simulink model "Quadrotor_1"  (R2018a)
settings: Solver=VariableStepAuto  StartTime=0.0  StopTime=100  MaxStep=0.001  RelTol=1e-3
settings Model: Creator=oussa  LastModifiedBy=oussa

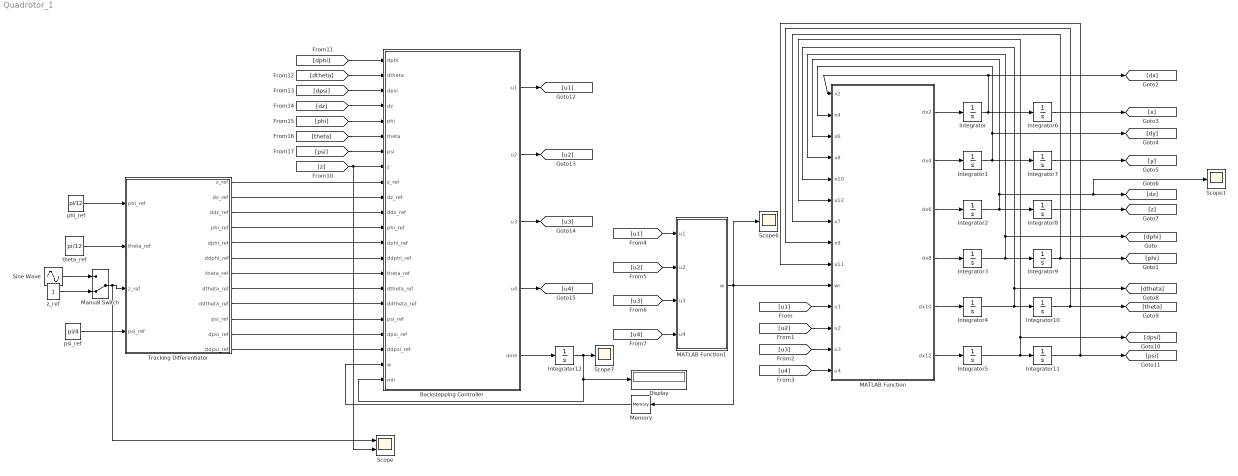
== system Quadrotor_1 ==
  Backstepping Controller : MATLAB Function  TreatAsAtomicUnit=on
  Display : Display
  Integrator{,1..11} (12 alike) : Integrator
  Integrator12 : Integrator  InitialCondition=0.01
  MATLAB Function : MATLAB Function  TreatAsAtomicUnit=on
  MATLAB Function1 : MATLAB Function  TreatAsAtomicUnit=on
  Manual Switch : ManualSwitch  CurrentSetting=0
  Memory : Memory  InitialCondition=500
  Scope : Scope  NumInputPorts=2
  Scope1 : Scope
  Scope6 : Scope
  Scope7 : Scope
  Sine Wave : Sin  SampleTime=0
  Tracking Differentiator : Subsystem
  phi_ref : Constant  Value=pi/12
  psi_ref : Constant  Value=pi/4
  theta_ref : Constant  Value=pi/12
  z_ref : Constant
  wires:
  MATLAB Function/1(dx2) -> Integrator/1
  MATLAB Function/2(dx4) -> Integrator1/1
  MATLAB Function/3(dx6) -> Integrator2/1
  MATLAB Function/4(dx8) -> Integrator3/1
  MATLAB Function/5(dx10) -> Integrator4/1
  MATLAB Function/6(dx12) -> Integrator5/1
  Integrator/1 -> MATLAB Function/1(x2), [dx], Integrator6/1
  Integrator1/1 -> [dy], MATLAB Function/2(x4), Integrator7/1
  Integrator3/1 -> [dphi], MATLAB Function/4(x8), Integrator9/1
  Integrator4/1 -> [dtheta], MATLAB Function/5(x10), Integrator10/1
  Integrator5/1 -> [dpsi], MATLAB Function/6(x12), Integrator11/1
  Integrator9/1 -> [phi], MATLAB Function/7(x7)
  Integrator10/1 -> [theta], MATLAB Function/8(x9)
  Integrator11/1 -> [psi], MATLAB Function/9(x11)
  MATLAB Function1/1(w) -> Memory/1, Scope6/1, MATLAB Function/10(wr)
  Backstepping Controller/3(u3) -> [u3]
  [psi] -> Backstepping Controller/7(psi)
  Backstepping Controller/4(u4) -> [u4]
  theta_ref/1 -> Tracking Differentiator/2(theta_ref)
  Backstepping Controller/2(u2) -> [u2]
  [dpsi] -> Backstepping Controller/3(dpsi)
  psi_ref/1 -> Tracking Differentiator/4(psi_ref)
  Backstepping Controller/5(dmh) -> Integrator12/1
  phi_ref/1 -> Tracking Differentiator/1(phi_ref)
  [dtheta] -> Backstepping Controller/2(dtheta)
  Backstepping Controller/1(u1) -> [u1]
  [theta] -> Backstepping Controller/6(theta)
  Tracking Differentiator/1("z_ref ") -> Backstepping Controller/9(z_ref)
  [phi] -> Backstepping Controller/5(phi)
  z_ref/1 -> Manual Switch/2
  Tracking Differentiator/7("theta_ref ") -> Backstepping Controller/15(theta_ref)
  Tracking Differentiator/9(ddtheta_ref) -> Backstepping Controller/17(ddtheta_ref)
  Tracking Differentiator/12(ddpsi_ref) -> Backstepping Controller/20(ddpsi_ref)
  Tracking Differentiator/5(dphi_ref) -> Backstepping Controller/13(dphi_ref)
  Manual Switch/1 -> Scope/1, Tracking Differentiator/3(z_ref)
  [z] -> Backstepping Controller/8(z), Scope/2
  Tracking Differentiator/11(dpsi_ref) -> Backstepping Controller/19(dpsi_ref)
  [dz] -> Backstepping Controller/4(dz)
  Tracking Differentiator/10("psi_ref ") -> Backstepping Controller/18(psi_ref)
  Tracking Differentiator/3(ddz_ref) -> Backstepping Controller/11(ddz_ref)
  Tracking Differentiator/8("dtheta_ref ") -> Backstepping Controller/16(dtheta_ref)
  Tracking Differentiator/4("phi_ref ") -> Backstepping Controller/12(phi_ref)
  Tracking Differentiator/2(dz_ref) -> Backstepping Controller/10(dz_ref)
  Tracking Differentiator/6(ddphi_ref) -> Backstepping Controller/14(ddphi_ref)
  [u1] -> MATLAB Function/11(u1)
  [u2] -> MATLAB Function/12(u2)
  [u3] -> MATLAB Function/13(u3)
  [u4] -> MATLAB Function/14(u4)
  [u1] -> MATLAB Function1/1(u1)
  [u2] -> MATLAB Function1/2(u2)
  [u3] -> MATLAB Function1/3(u3)
  [u4] -> MATLAB Function1/4(u4)
  Integrator6/1 -> [x]
  Integrator7/1 -> [y]
  Integrator8/1 -> [z]
  [dphi] -> Backstepping Controller/1(dphi)
  Integrator12/1 -> Display/1, Backstepping Controller/22(mh), Scope7/1
  Memory/1 -> Backstepping Controller/21(w)
  Integrator2/1 -> Scope1/1, [dz], MATLAB Function/3(x6), Integrator8/1
  Sine Wave/1 -> Manual Switch/1

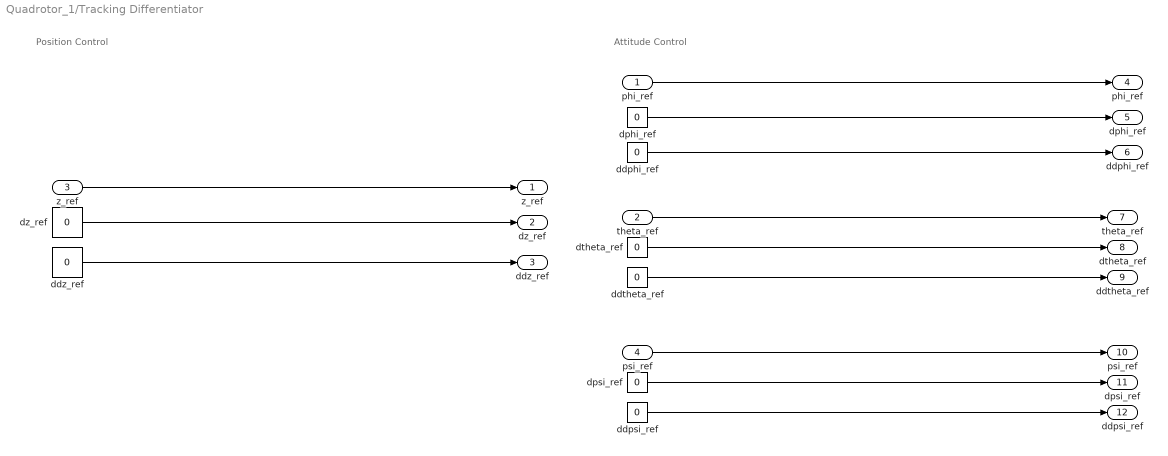
== system Quadrotor_1/Tracking Differentiator ==
  note: Attitude Control
  note: Position Control
  phi_ref : Inport
  theta_ref : Inport  Port=2
  z_ref : Inport  Port=3
  psi_ref : Inport  Port=4
  "ddphi_ref " : Constant  Value=0
  "ddpsi_ref " : Constant  Value=0
  "ddtheta_ref " : Constant  Value=0
  "ddz_ref " : Constant  Value=0
  "dphi_ref " : Constant  Value=0
  "dpsi_ref " : Constant  Value=0
  dtheta_ref : Constant  Value=0
  "dz_ref " : Constant  Value=0
  "z_ref " : Outport
  dz_ref : Outport  Port=2
  ddz_ref : Outport  Port=3
  "phi_ref " : Outport  Port=4
  dphi_ref : Outport  Port=5
  ddphi_ref : Outport  Port=6
  "theta_ref " : Outport  Port=7
  "dtheta_ref " : Outport  Port=8
  ddtheta_ref : Outport  Port=9
  "psi_ref " : Outport  Port=10
  dpsi_ref : Outport  Port=11
  ddpsi_ref : Outport  Port=12
  wires:
  phi_ref/1 -> "phi_ref "/1
  theta_ref/1 -> "theta_ref "/1
  psi_ref/1 -> "psi_ref "/1
  z_ref/1 -> "z_ref "/1
  "dz_ref "/1 -> dz_ref/1
  "ddz_ref "/1 -> ddz_ref/1
  "dphi_ref "/1 -> dphi_ref/1
  "ddphi_ref "/1 -> ddphi_ref/1
  dtheta_ref/1 -> "dtheta_ref "/1
  "ddtheta_ref "/1 -> ddtheta_ref/1
  "ddpsi_ref "/1 -> ddpsi_ref/1
  "dpsi_ref "/1 -> dpsi_ref/1

== matlab function Quadrotor_1/MATLAB Function1 ==
  data: u1 input; w output; u2 input; u3 input; u4 input
function w = fcn(u1,u2,u3,u4)

b = 2.9e-5;
d = 1.1e-6;
l = 0.21;

A = [b b b b;0 l*b 0 -l*b;l*b 0 -l*b 0;d -d d -d];

 wr = pinv(A)*[u1;u2;u3;u4];

    for i=1:4
       if wr(i)<0
           wr(i) = 0;
       end
    end
  
 w = sqrt(wr(4))-sqrt(wr(3))+sqrt(wr(2))-sqrt(wr(1));

== matlab function Quadrotor_1/MATLAB Function ==
  data: x2 input; dx2 output; x4 input; x6 input; x8 input; x10 input; x12 input; x7 input; x9 input; x11 input; wr input; u1 input; u2 input; u3 input; u4 input; dx4 output; dx6 output; dx8 output; dx10 output; dx12 output
function [dx2,dx4,dx6,dx8,dx10,dx12] = Quadrotor_Model(x2,x4,x6,x8,x10,x12,x7,x9,x11,wr,u1,u2,u3,u4)

m = 0.74;
Ix = 0.004;
Iy = Ix;
Iz = 0.0084;
g = 9.81;
kx = 5.567e-5;
ky = kx;
kz = ky;
kphi = 5.567e-5;
ktht = kphi;
kpsi = ktht;
Jr = 2.838e-5;

a1 = (Iy-Iz)/Ix; a2 = -Jr/Ix; a3 = -kphi/Ix;
b1 = (Iz-Ix)/Iy; b2 = Jr/Iy;  b3 = -ktht/Iy;
c1 = (Ix-Iy)/Iz; c2 = -kpsi/Iz;


dx2 = (sin(x7)*sin(x11)+cos(x11)*cos(x7)*sin(x9))*u1/m-kx/m*abs(x2)*x2;
dx4 = (cos(x7)*sin(x9)*sin(x11)-sin(x7)*cos(x11))*u1/m-ky/m*abs(x4)*x4;
dx6 = -g+(cos(x7)*cos(x9))/m*u1-kz/m*abs(x6)*x6;

dx8 = a1*x10*x12+a2*wr*x10+a3*x8^2+1/Ix*u2;
dx10 = b1*x8*x12+b2*wr*x8+b3*x10^2+1/Iy*u3;
dx12 = c1*x8*x10+c2*x12^2+1/Iz*u4;

== matlab function Quadrotor_1/Backstepping Controller ==
  data: dphi input; dtheta input; dpsi input; dz input; phi input; theta input; psi input; z input; z_ref input; dz_ref input; ddz_ref input; phi_ref input; dphi_ref input; ddphi_ref input; theta_ref input; dtheta_ref input; u1 output; u2 output; u3 output; u4 output; ddtheta_ref input; psi_ref input; dpsi_ref input; ddpsi_ref input; w input; mh input size=1; dmh output size=1
function [u1,u2,u3,u4,dmh] = Backstepping_Controller(dphi,dtheta,dpsi,dz,phi,theta,psi,z,z_ref,dz_ref,ddz_ref,phi_ref,dphi_ref,ddphi_ref,theta_ref,dtheta_ref,ddtheta_ref,psi_ref,dpsi_ref,ddpsi_ref,w,mh)


Ix = 0.004;
Iy = 0.004;
Iz = 0.0084;
Ir = 2.8385e-5;
g = 9.81;
L = 0.225;
kz = 1e-3;
kphi = 1e-2;
ktheta = 1e-2;
kpsi = 1e-2;
gama = 0.1;

a1 = (Iy-Iz)/Ix; a2 = -Ir/Ix; b1 = L/Ix;
a3 = (Iz-Ix)/Iy; a4 = Ir/Iy; b2 = L/Iy;
a5= (Ix-Iy)/Iz; b3 = 1/Iz;



k1 = 2;
k2 = 10;
k3 = 2;
k4 = 10;
k5 = 2;
k6 = 10;
k7 = 0.5;
k8 = 1;

e1 = phi_ref-phi;
e2 = dphi-k1*e1-dphi_ref;
u2 = 1/b1*(-k2*e2+e1+ddphi_ref-k1*(e2+k1*e1)-a1*dtheta*dpsi-a2*dtheta*w+kphi/Ix*dphi*abs(dphi));

e3 = theta_ref-theta;
e4 = dtheta-dtheta_ref-k3*e3;
u3 = 1/b2*(-k4*e4+e3-a3*dphi*dpsi-a4*w*dphi+ddtheta_ref-k3*(e4+k3*e3)+ktheta/Iy*dtheta*abs(dtheta));

e5 = psi_ref-psi;
e6 = dpsi-dpsi_ref-k5*e5;
u4 = 1/b3*(-k6*e6+e5-a5*dphi*dtheta+ddpsi_ref-k5*(e6+k5*e5)+kpsi/Iz*dpsi*abs(dpsi));


e7 = z_ref-z;
de7 = -dz+dz_ref;
e8 = dz-dz_ref-k7*e7;
dmh = -gama*(g+e7-k8*e8+k7*de7+ddz_ref)*e8;
u1 = mh/(cos(phi)*cos(theta))*(-k8*e8+e7+g-k7*(e8+k7*e7)+ddz_ref+kz/mh*dz);

end
